simulink model "ImplementTestHarness"  (R2024b)
settings: Solver=daessc  StartTime=0.0  StopTime=10.0  RelTol=1e-3
libraries: fl_lib x6, nesl_utility x4, SignalEditorBlockLib x1
settings Model: Creator=asakhare  LastModifiedBy=varora
settings SolverCC: MaxConsecutiveZCs=10  MaxConsecutiveMinStep=10
settings SimscapeCC: SimscapeLogType=all

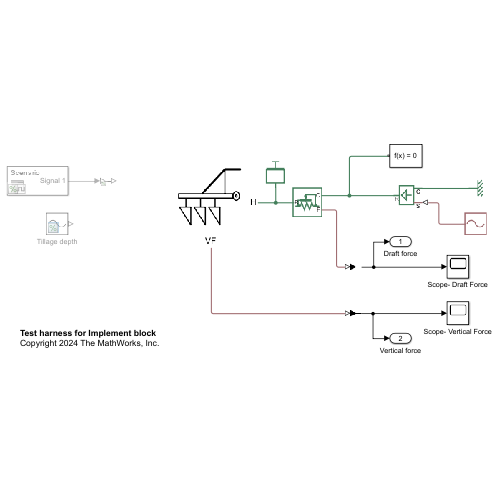
[thumbnail: Simulink's stored preview of the top-level diagram]
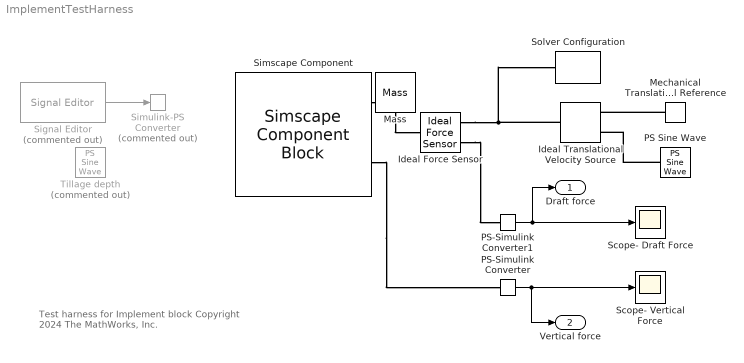
== system ImplementTestHarness ==
  note: Test harness for Implement block
      | Copyright 2024 The MathWorks, Inc.
  Ideal Force Sensor : fl_lib/Mechanical/Mechanical Sensors/Ideal Force Sensor
  Ideal Translational Velocity Source : fl_lib/Mechanical/Mechanical Sources/Ideal Translational Velocity Source
  Mass : fl_lib/Mechanical/Translational Elements/Mass  mass=1 kg  num_ports=foundation.enum.numPorts2.one  v_specify=off  v_priority=High  v=0 m/s  v_nominal_specify=off  v_nominal_value=1  v_nominal_unit=m/s  f_specify=off  f_priority=None  f=0 N  f_nominal_specify=off  f_nominal_value=1  f_nominal_unit=N
  Mechanical Translational Reference : fl_lib/Mechanical/Translational Elements/Mechanical Translational Reference
  PS Sine Wave : fl_lib/Physical Signals/Sources/PS Sine Wave  amplitude=3 m/s  bias=0 m/s  frequency_spec=foundation.enum.frequencySpec.frequencySI  frequency_SI=1/10 Hz  frequency_angular=1 rad/s  phase=0 rad
      settings: InternalSimscapePortConfiguration="{\"Bottom\":[],\"Left\":[],\"Right\":[{\"id\":\"O\",\"label\":\"\",\"type\":\"output\"}],\"Top\":[]}"
  PS-Simulink Converter : nesl_utility/PS-Simulink Converter  PhysicalDomain=network_engine_domain  SubClassName=ps_output  LeftPortType=input  RightPortType=output  PseudoPeriodic=off  Frequencies=[]  VectorFormat=inherit  Unit=N  AffineConversion=off
  PS-Simulink Converter1 : nesl_utility/PS-Simulink Converter  PhysicalDomain=network_engine_domain  SubClassName=ps_output  LeftPortType=input  RightPortType=output  PseudoPeriodic=off  Frequencies=[]  VectorFormat=inherit  Unit=N  AffineConversion=off
  Scope- Draft Force : Scope
  Scope- Vertical Force : Scope
  Signal Editor : SignalEditorBlockLib/Signal Editor  Commented=on  FileName=soilTextureSignal.mat  ActiveScenario=Scenario  ActiveSignal=Signal 1  IsBus=off  OutputBusObjectStr=Bus: BusObject  SampleTime=0  Interpolate=off  ZeroCross=off  OutputAfterFinalValue=Setting to zero  Unit=inherit  PreserveSignalName=on  ApplySigPropsToAllScenarios=on  ApplySigPropsToAllSignals=off
  Simscape Component : SimscapeComponentBlock  SourceFile=implement  ComponentPath=implement  ComponentVariants="[\"implement\"]"  ComponentVariantNames="[\"implement\"]"  ClassName=implement  SchemaVersion=1  parameterization=ForceComputation.UserInput  type_implement=ImplementType.Subsoiler  width_implement=1 m  number_tools=5  rake_angle=45 deg  velocity_vector=[-2,-1, 0, 1, 2] m/s  draft_vector=[-2000, -1000, 0, 1000, 2000] N  VF_vector=[600, 300, 0, 300, 600] N  velocity_thr=1e-6 m/s  depth_min=1e-6 cm
      settings: CopyFcn=simscape.engine.sli.internal.componentblockcallback(gcbh,'COPY')  PreCopyFcn=simscape.engine.sli.internal.componentblockcallback(gcbh,'PRECOPY')  PreDeleteFcn=simscape.engine.sli.internal.componentblockcallback(gcbh,'PREDELETE')  InternalSimscapePortConfiguration="{\"Bottom\":[{\"id\":\"VF\",\"label\":\"VF\",\"type\":\"output\"}],\"Left\":[],\"Right\":[{\"id\":\"H\",\"label\":\"H\",\"type\":\"foundation.mechanical.translational.translational\"}],\"Top\":[]}"
      mask Type: Implement
  Simulink-PS Converter : nesl_utility/Simulink-PS Converter  Commented=on  PhysicalDomain=network_engine_domain  SubClassName=ps_input  LeftPortType=input  RightPortType=output  PseudoPeriodic=off  Frequencies=[]  NoiseDistribution=none  NoiseParameters=[]  Unit=1  AffineConversion=off  FilteringAndDerivatives=provide  SimscapeFilterOrder=1  InputFilterTimeConstant=0.001  UdotUserProvided=0
  Solver Configuration : nesl_utility/Solver Configuration  PhysicalDomain=network_engine_domain  SubClassName=solver  LeftPortType=input  RightPortType=generic  Tones=[]  Harmonics=[]  SimulateNoise=off  Profile=off  UseLocalSampling=off  EnableSwitchedLinearOptims=on  FrequencyDomain=off  UseCCode=off  RelTol=0.001  AbsTol=0.001  MinStep=1e-09  ToWorkspace=off  RevertToSquareIcSolve=off  NumHomotopyIterations=100  PhasorMode=off  PhasorModeNumHarmonics=1  ConsistencySolver=NEWTON_XTOL_AFTER_FTOL  IndexReductionMethod=DerivativeReplacement  DoDC=off  ResidualTolerance=1e-09  ConsistencyTolSource=GLOBAL  ConsistencyAbsTol=0.001  ConsistencyRelTol=0.001  ConsistencyTolFactor=0.001  UseLocalSolver=off  LocalSolverChoice=NE_BACKWARD_EULER_ADVANCER  ResolveIndetEquations=on  FunctionEvalNumThread=1  LocalSolverSampleTime=0.001  DoFixedCost=off  MaxNonlinIter=3  MaxModeIter=2  ComputeImpulses=off  ImpulseIterations=2  LinearAlgebra=auto  LinearAlgebraNumThread=0  EquationFormulation=NE_TIME_EF  DelaysMemoryBudget=1024  AutomaticFiltering=on  FilteringTimeConstant=0.001  PartitionStorageMethod=AS_NEEDED  PartitionMemoryBudget=1024  PartitionMethod=ROBUST  MultibodyUseLocalSolver=off  MultibodyLocalSolverChoice=ODE1  MultibodyLocalSolverSampleTime=0.001
  Tillage depth : fl_lib/Physical Signals/Sources/PS Sine Wave  Commented=on  amplitude=1 cm  bias=0.5 cm  frequency_spec=foundation.enum.frequencySpec.frequencySI  frequency_SI=1/10 Hz  frequency_angular=1 rad/s  phase=pi/2 rad
      settings: InternalSimscapePortConfiguration="{\"Bottom\":[],\"Left\":[],\"Right\":[{\"id\":\"O\",\"label\":\"\",\"type\":\"output\"}],\"Top\":[]}"
  Draft force : Outport
  Vertical force : Outport  Port=2
  wires:
  PS-Simulink Converter/1 -> Scope- Vertical Force/1, Vertical force/1
  Signal Editor/1 -> Simulink-PS Converter/1
  PS-Simulink Converter1/1 -> Scope- Draft Force/1, Draft force/1
  connections:
  Simscape Component/RConn2 -- PS-Simulink Converter/LConn1
  Mechanical Translational Reference/LConn1 -- Ideal Translational Velocity Source/RConn2
  PS Sine Wave/RConn1 -- Ideal Translational Velocity Source/RConn1
  Simscape Component/RConn1 -- Mass/LConn1 -- Ideal Force Sensor/LConn1
  Ideal Force Sensor/RConn2 -- PS-Simulink Converter1/LConn1
  Ideal Translational Velocity Source/LConn1 -- Solver Configuration/RConn1 -- Ideal Force Sensor/RConn1
